simulink model "Draw_U"  (R2018a)
settings: Solver=VariableStepAuto  StartTime=0.0  StopTime=1.6  MaxStep=0.01  RelTol=1e-3  EnableMultiTasking=on
model workspace: external: MATLAB File D:\Google Drive\Duongw_Folder\Thesis Master\_Model\Delta_Model_ADEPT\SIMCAPE_MULTI_BODY\ADEPT_DELTA_3AXES1\Assem1_ADEPT_HORNET_DataFile.m (data not in the file)
values from neighbouring files (symbols this model uses):
  m = zeros(1,3)    [forward.m]    (also in solequa.m = zeros(3,1))
  smiData = struct    [Assem1_ADEPT_HORNET_DataFile.m]
undefined symbols (not defined in the file or in its folder): X, Y, Z
libraries: sm_lib x106, nesl_utility x7
(part 3 of 3)

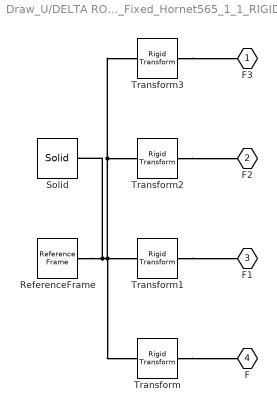
== system Draw_U/DELTA ROBOT MODEL/Platform_Fixed_Hornet565_1_1_RIGID ==
  ReferenceFrame : sm_lib/Frames and Transforms/Reference Frame
  Solid : sm_lib/Body Elements/Solid  InertiaType=Custom  Mass=0.4  MassUnits=kg  CenterOfMass=smiData.Solid(5).CoM  CenterOfMassUnits=mm  MomentsOfInertia=smiData.Solid(5).MoI  MomentsOfInertiaUnits=kg*mm^2  ProductsOfInertia=smiData.Solid(5).PoI  ProductsOfInertiaUnits=kg*mm^2  DensityBased=on  Density=1000  DensityUnits=kg/(m^3)  DoExposeReferenceFrame=on  SerializedFrames=<Frames/>  GraphicType=FromGeometry  MarkerShape=Sphere  MarkerSize=10  GraphicVisPropType=SimpleVisualProperties  GraphicDiffuseColor=smiData.Solid(5).color  GraphicSpecularColor=[0.5 0.5 0.5 1.0]  GraphicAmbientColor=[0.15 0.15 0.15 1.0]  GraphicEmissiveColor=[0.0 0.0 0.0 1.0]  GraphicShininess=75  GraphicOpacity=smiData.Solid(5).opacity  GeometryShape=FromFile  RectangleSize=[1 1]  RectangleSizeUnits=m  BrickDimensions=[1 1 1]  BrickDimensionUnits=m  CylinderRadius=1  CylinderRadiusUnits=m  CylinderLength=1  CylinderLengthUnits=m  SphereRadius=1  SphereRadiusUnits=m  EllipsoidRadii=[1 1 1]  EllipsoidRadiiUnits=m  ExtrusionCrossSection=[1 1; -1 1; -1 -1; 1 -1]  ExtrusionCrossSectionUnits=m  ExtrusionLength=1  ExtrusionLengthUnits=m  PolygonNumSides=3  PolygonOuterRadius=1  PolygonOuterRadiusUnits=m  ExtGeomFileType=STEP  ExtGeomFileName=Platform_Fixed-Hornet565_1_Default_sldprt.STEP  ExtGeomFileUnits=m  RevolutionCrossSection=[1 1; 1 -1; 2 -1; 2 1]  RevolutionCrossSectionUnits=m  RevolutionExtent=Full  RevolutionAngle=180  RevolutionAngleUnits=deg
  Transform : sm_lib/Frames and Transforms/Rigid Transform  TranslationMethod=Cartesian  TranslationStandardOffset=0  TranslationLengthUnit=mm  TranslationStandardAxis=+Z  TranslationCartesianOffset=smiData.RigidTransform(1).translation  TranslationROffset=0  TranslationROffsetUnits=m  TranslationZOffset=0  TranslationZOffsetUnits=m  TranslationThetaOffset=0  TranslationThetaOffsetUnits=deg  RotationMethod=ArbitraryAxis  RotationAngleUnits=rad  RotationStandardAxis=+Z  RotationAngle=smiData.RigidTransform(1).angle  RotationArbitraryAxis=smiData.RigidTransform(1).axis  FollAlignAxisA=+X  BaseAlignAxisA=+Y  FollAlignAxisB=+Y  BaseAlignAxisB=+Z  RotationSequenceAxes=FollowerAxes  RotationSequence=XYX  RotationSequenceAngles=[0 0 0]  RotationSequenceAnglesUnits=deg  RotationMatrix=[1 0 0; 0 1 0; 0 0 1]
  Transform1 : sm_lib/Frames and Transforms/Rigid Transform  TranslationMethod=Cartesian  TranslationStandardOffset=0  TranslationLengthUnit=mm  TranslationStandardAxis=+Z  TranslationCartesianOffset=smiData.RigidTransform(32).translation  TranslationROffset=0  TranslationROffsetUnits=m  TranslationZOffset=0  TranslationZOffsetUnits=m  TranslationThetaOffset=0  TranslationThetaOffsetUnits=deg  RotationMethod=ArbitraryAxis  RotationAngleUnits=rad  RotationStandardAxis=+Z  RotationAngle=smiData.RigidTransform(32).angle  RotationArbitraryAxis=smiData.RigidTransform(32).axis  FollAlignAxisA=+X  BaseAlignAxisA=+Y  FollAlignAxisB=+Y  BaseAlignAxisB=+Z  RotationSequenceAxes=FollowerAxes  RotationSequence=XYX  RotationSequenceAngles=[0 0 0]  RotationSequenceAnglesUnits=deg  RotationMatrix=[1 0 0; 0 1 0; 0 0 1]
  Transform2 : sm_lib/Frames and Transforms/Rigid Transform  TranslationMethod=Cartesian  TranslationStandardOffset=0  TranslationLengthUnit=mm  TranslationStandardAxis=+Z  TranslationCartesianOffset=smiData.RigidTransform(38).translation  TranslationROffset=0  TranslationROffsetUnits=m  TranslationZOffset=0  TranslationZOffsetUnits=m  TranslationThetaOffset=0  TranslationThetaOffsetUnits=deg  RotationMethod=ArbitraryAxis  RotationAngleUnits=rad  RotationStandardAxis=+Z  RotationAngle=smiData.RigidTransform(38).angle  RotationArbitraryAxis=smiData.RigidTransform(38).axis  FollAlignAxisA=+X  BaseAlignAxisA=+Y  FollAlignAxisB=+Y  BaseAlignAxisB=+Z  RotationSequenceAxes=FollowerAxes  RotationSequence=XYX  RotationSequenceAngles=[0 0 0]  RotationSequenceAnglesUnits=deg  RotationMatrix=[1 0 0; 0 1 0; 0 0 1]
  Transform3 : sm_lib/Frames and Transforms/Rigid Transform  TranslationMethod=Cartesian  TranslationStandardOffset=0  TranslationLengthUnit=mm  TranslationStandardAxis=+Z  TranslationCartesianOffset=smiData.RigidTransform(44).translation  TranslationROffset=0  TranslationROffsetUnits=m  TranslationZOffset=0  TranslationZOffsetUnits=m  TranslationThetaOffset=0  TranslationThetaOffsetUnits=deg  RotationMethod=ArbitraryAxis  RotationAngleUnits=rad  RotationStandardAxis=+Z  RotationAngle=smiData.RigidTransform(44).angle  RotationArbitraryAxis=smiData.RigidTransform(44).axis  FollAlignAxisA=+X  BaseAlignAxisA=+Y  FollAlignAxisB=+Y  BaseAlignAxisB=+Z  RotationSequenceAxes=FollowerAxes  RotationSequence=XYX  RotationSequenceAngles=[0 0 0]  RotationSequenceAnglesUnits=deg  RotationMatrix=[1 0 0; 0 1 0; 0 0 1]
  F3 : PMIOPort  Side=Left
  F2 : PMIOPort  Port=2  Side=Left
  F1 : PMIOPort  Port=3  Side=Left
  F : PMIOPort  Port=4  Side=Right
  connections:
  Solid/RConn1 -- ReferenceFrame/RConn1 -- Transform2/LConn1 -- Transform3/LConn1 -- Transform/LConn1 -- Transform1/LConn1
  Transform/RConn1 -- F/RConn1
  Transform1/RConn1 -- F1/RConn1
  Transform2/RConn1 -- F2/RConn1
  Transform3/RConn1 -- F3/RConn1

== matlab function Draw_U/U_Path_Trajectory  ==
  data: x output; t input; y output; z output
function [x,y,z] = fcn(t)
to = 0; tf = 1.6; % Thoi gian chuyen dong
t1 = 0.4;t2=0.8;t3 = 1.2; % Cac thoi diem chuyen tiep
xo =0; yo = 0; zo = 0.85;
xe =0.4; ye =0.3; ze = 0.65;
x = 0*t;
y = 0*t;
z = 0*t;
% Tinh ma tran Cz2
Az2 = [ze;zo;0;0;0;0];
Bz2 = [t2^5 t2^4 t2^3 t2^2 t2 1; tf^5 tf^4 tf^3 tf^2 tf 1; 5*t2^4 4*t2^3 3*t2^2 2*t2 1 0; 5*tf^4 4*tf^3 3*tf^2 2*tf 1 0; 20*t2^3 12*t2^2 6*t2 2 0 0; 20*tf^3 12*tf^2 6*tf 2 0 0];
Cz2 = Bz2\Az2;% ma tran he so da thuc quy dao tu t2 den tf
%Tinh ma tran Cz1
Az1 = [zo;ze;0;0;0;0];
Bz1 = [to^5 to^4 to^3 to^2 to 1; t2^5 t2^4 t2^3 t2^2 t2 1; 5*to^4 4*to^3 3*to^2 2*to 1 0; 5*t2^4 4*t2^3 3*t2^2 2*t2 1 0; 20*to^3 12*to^2 6*to 2 0 0; 20*t2^3 12*t2^2 6*t2 2 0 0];
Cz1 = Bz1\Az1;% ma tran he so da thuc quy dao tu t0 den t2

%Quy dao theo toa do z
   if (to<=t)&&(t<=t2) % Quy dao tu t0 den t2
       z= Cz1(1)*t^5+Cz1(2)*t^4+Cz1(3)*t^3+Cz1(4)*t^2+Cz1(5)*t+Cz1(6);
   end
   if (t2<=t)&&(t<=tf) % Quy dao tu t2 den tf
       z= Cz2(1)*t^5+Cz2(2)*t^4+Cz2(3)*t^3+Cz2(4)*t^2+Cz2(5)*t+Cz2(6);
   end
%Xay dung quy dao toa do x
Ax = [xo;xe;0;0;0;0];
Bx = [t1^5 t1^4 t1^3 t1^2 t1 1; t3^5 t3^4 t3^3 t3^2 t3 1; 5*t1^4 4*t1^3 3*t1^2 2*t1 1 0; 5*t3^4 4*t3^3 3*t3^2 2*t3 1 0; 20*t1^3 12*t1^2 6*t1 2 0 0; 20*t3^3 12*t3^2 6*t3 2 0 0];
Cx = Bx\Ax;% ma tran he so da thuc quy dao tu t1 den t3
%Quy dao toa do x
    if (to<=t)&&(t<=t1)
        x = 0;
    end
    if(t1<=t)&&(t<=t3)
        x= Cx(1)*t^5+Cx(2)*t^4+Cx(3)*t^3+Cx(4)*t^2+Cx(5)*t+Cx(6);
    end
    if(t3<=t)&&(t<=tf)
       x = 0.4; 
    end
y = (ye-yo)/(xe-xo)*x;

== matlab function Draw_U/Invert_Kinematics/MATLAB Function ==
  data: x input; theta1 output; y input; z input; theta2 output; theta3 output
function [theta1, theta2, theta3] = fcn(x,y,z)
%Ham giai bai toan dong hoc nguoc
%phuong trinh dong hoc nguoc : a*cos(theta)+b*sin(theta) = c
r1 = 0.225; % Radius of circle crosses three revolute joints of the Base
r2 = 0.075;  % Radius of circle crosses three revolute joints of the Moving platform
r = r2 - r1;
l1 = 0.315;         % Kinematics Length of Active arms
l2 = 0.825;         % Kinematics length of Driven arms
phi1 = pi/2;
phi2 = 7*pi/6;
phi3 = 11*pi/6;
phi = [phi1; phi2; phi3];
%--------------------------------------------------------------------------
    a1 = 2*l1*(r+x*cos(phi(1))+y*sin(phi(1)));
    b1 = 2*z*l1;
    c1 = x^2 + y^2 + z^2 + r^2 +l1^2-l2^2+2*r*(y*sin(phi(1))+x*cos(phi(1)));
    anfa1 = asin(a1/(sqrt(a1^2+b1^2)));
    theta1 = asin(c1/(sqrt(a1^2+b1^2)))- anfa1;
%--------------------------------------------------------------------------
    a2 = 2*l1*(r+x*cos(phi(2))+y*sin(phi(2)));
    b2 = 2*z*l1;
    c2 = x^2 + y^2 + z^2 + r^2 +l1^2-l2^2+2*r*(y*sin(phi(2))+x*cos(phi(2)));
    anfa2 = asin(a2/(sqrt(a2^2+b2^2)));
    theta2 = asin(c2/(sqrt(a2^2+b2^2)))- anfa2;
%--------------------------------------------------------------------------
    a3 = 2*l1*(r+x*cos(phi(3))+y*sin(phi(3)));
    b3 = 2*z*l1;
    c3 = x^2 + y^2 + z^2 + r^2 +l1^2-l2^2+2*r*(y*sin(phi(3))+x*cos(phi(3)));
    anfa3 = asin(a3/(sqrt(a3^2+b3^2)));
    theta3 = asin(c3/(sqrt(a3^2+b3^2)))- anfa3;
